simulink model "PMSM3P2LInverterCHILsystem"  (R2026a)
settings: Solver=FixedStepAuto  StopTime=inf  FixedStep=Ts_CPU  EnableMultiTasking=on
undefined symbols (not defined in the file): DiscIntNeverNeededParam, F28379D_ADC_MaxCount, F28379D_ADC_Vmax, Foc_Ki_IxTcpu, Foc_Ki_S, Foc_Kp_I, Foc_Kp_S, Ia_offset, Ib_offset, IO334, IO334_DAC_Vmax, IO334_iDAC_bias, IO334_iDAC_gain, Maxon_645604_J, Maxon_645604_lambda_pm, Maxon_645604_Ld, Maxon_645604_Lq, Maxon_645604_Np, Maxon_645604_Rs, Maxon_645604_StaticF, Maxon_645604_ViscousF, Maxon_Mile_Nslits, PMSM3P2LInverter_limited, PMSM_3P2L_Inverter_Plant, PU_System_I_base, PU_System_N_base, PWM_frequency, Ts_CAN_Tx, Ts_CPU, ts_FPGA_mdl, Ts_UI
libraries: speedgoatlib_hdlCoder_IO3xx x31, mcbcontrolslib x8, canmsglib x6, speedgoatlib_IO611 x3, mcbeeMathTransformLib x3, slpidlib x3, simulink x3, mcbpositiondecoderlib x3, pwm_cpulib x2, mcbhdlplantlib x2, demo_controls x1, quadrature_cpulib x1
(part 2 of 3)

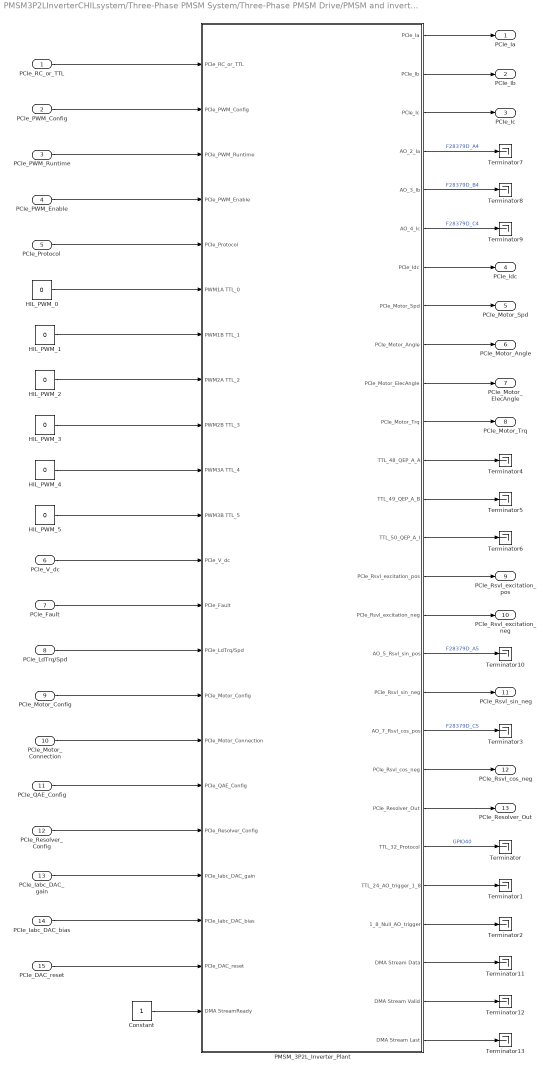
== system PMSM3P2LInverterCHILsystem/Three-Phase PMSM System/Three-Phase PMSM Drive/PMSM and inverter with switching dynamics/PMSM_3P2L_Inverter_Plant_TBR ==
  PCIe_RC_or_TTL : Inport
  PCIe_PWM_Config : Inport  Port=2
  PCIe_PWM_Runtime : Inport  Port=3
  PCIe_PWM_Enable : Inport  Port=4
  PCIe_Protocol : Inport  Port=5
  PCIe_V_dc : Inport  Port=6
  PCIe_Fault : Inport  Port=7
  PCIe_LdTrq/Spd : Inport  Port=8
  PCIe_Motor_Config : Inport  Port=9
  PCIe_Motor_Connection : Inport  Port=10
  PCIe_QAE_Config : Inport  Port=11
  PCIe_Resolver_Config : Inport  Port=12
  PCIe_Iabc_DAC_gain : Inport  Port=13
  PCIe_Iabc_DAC_bias : Inport  Port=14
  PCIe_DAC_reset : Inport  Port=15
  Constant : Constant  OutDataTypeStr=boolean
  HIL_PWM_{0..5} (6 alike) : Constant  Value=0  OutDataTypeStr=boolean
  PMSM_3P2L_Inverter_Plant : Subsystem  mask(Speedgoat IO334-325k Interface Block){module_id=1, slot=-1, ts=-1, dacGain_1=+/- 10.0V, dacActiv_1=off, dacGain_2=+/- 2.5V, dacActiv_2=on, dacGain_3=+/- 2.5V, dacActiv_3=on, dacGain_4=+/- 2.5V, dacActiv_4=on, dacGain_5=+/- 2.5V, dacActiv_5=on, dacGain_6=+/- 10.0V, dacActiv_6=off, dacGain_7=+/- 2.5V, dacActiv_7=on, dacGain_8=+/- 10.0V, dacActiv_8=off, dacGain_9=+/- 10.0V, dacActiv_9=off, dacGain_10=+/- 10.0V, dacActiv_10=off, dacGain_11=+/- 10.0V, dacActiv_11=off, dacGain_12=+/- 10.0V, dacActiv_12=off, dacGain_13=+/- 10.0V, dacActiv_13=off, dacGain_14=+/- 10.0V, dacActiv_14=off, dacGain_15=+/- 10.0V, dacActiv_15=off, dacGain_16=+/- 10.0V, dacActiv_16=off, PullRPort0=pull-up 3.3V, VioPort0=3.3V, PullRPort1=pull-up 3.3V, VioPort1=3.3V, PullRPort2=pull-up 3.3V, VioPort2=3.3V, PullRPort3=pull-up 3.3V, VioPort3=3.3V, PullRPort4=pull-up 3.3V, VioPort4=3.3V, PullRPort5=pull-up 3.3V, VioPort5=3.3V, PullRPort6=pull-up 3.3V, VioPort6=3.3V, fpga_sync_mode=on, reset_mode=on, reset_mode_stop=on, FpgaFreq=200}
      mask prompts: module_id "FPGA Module Identifier:"; slot "PCI slot (-1: autosearch):"; ts "Sample time:"; dacGain_1 "DAC Ch 01 Range"; dacActiv_1 "Active"; dacGain_2 "DAC Ch 02 Range"; dacActiv_2 "Active"; dacGain_3 "DAC Ch 03 Range"; dacActiv_3 "Active"; dacGain_4 "DAC Ch 04 Range"; dacActiv_4 "Active"; dacGain_5 "DAC Ch 05 Range"; dacActiv_5 "Active"; dacGain_6 "DAC Ch 06 Range"; dacActiv_6 "Active"; dacGain_7 "DAC Ch 07 Range"; dacActiv_7 "Active"; dacGain_8 "DAC Ch 08 Range"; dacActiv_8 "Active"; dacGain_9 "DAC Ch 09 Range"; dacActiv_9 "Active"; dacGain_10 "DAC Ch 10 Range"; dacActiv_10 "Active"; dacGain_11 "DAC Ch 11 Range"; dacActiv_11 "Active"; dacGain_12 "DAC Ch 12 Range"; dacActiv_12 "Active"; dacGain_13 "DAC Ch 13 Range"; dacActiv_13 "Active"; dacGain_14 "DAC Ch 14 Range"; dacActiv_14 "Active"; dacGain_15 "DAC Ch 15 Range"; dacActiv_15 "Active"; dacGain_16 "DAC Ch 16 Range"; dacActiv_16 "Active"; PullRPort0 "pull resistor"; VioPort0 "I/O voltage"; PullRPort1 "pull resistor"; VioPort1 "I/O voltage"; PullRPort2 "pull resistor"; VioPort2 "I/O voltage"; PullRPort3 "pull resistor"; VioPort3 "I/O voltage"; PullRPort4 "pull resistor"; VioPort4 "I/O voltage"; PullRPort5 "pull resistor"; VioPort5 "I/O voltage"; PullRPort6 "pull resistor"; VioPort6 "I/O voltage"; fpga_sync_mode "Run FPGA only when target application runs"; reset_mode "Reset FPGA states on start"; reset_mode_stop "Reset FPGA states on stop"; FpgaFreq "FPGA Frequency [MHz]"
      mask help: Simulink Real-Time Interface Block for Speedgoat IO334-325k.
      mask init:
      | hdlslrt.backend.mfpgaparameters;
      | if sg.hdlc.utils.compareMatlabVersion('~=', 'R2025a')
      | 	sg.hdlc.warning(['The interface model that you are attempting to use was generated ',...
      | 		'in MATLAB R2025a and may not be compatible with the version you are currently using. ',...
      | 		'Attempting to use this interface model in a different MATLAB release can lead to ',...
      | 		'application crashes or other unpredictable behavior. ',...
      | 		'In order to avoid this and ensure stability and correct functionality, ',...
      | 		'we highly recommend regenerating the model with your current MATLAB release.']);
      | end
      mask Help: eval('sg.hdlc.utils.help.show(''refentry_workflow_generated_model'',''isHdlcHelp'', true)')
      mask TypeOptions dacGain_1: AD5547 Setup/dacGain_1
      mask TypeOptions dacActiv_1: AD5547 Setup/dacActiv_1
      mask TypeOptions dacGain_2: AD5547 Setup/dacGain_2
      mask TypeOptions dacActiv_2: AD5547 Setup/dacActiv_2
      mask TypeOptions dacGain_3: AD5547 Setup/dacGain_3
      mask TypeOptions dacActiv_3: AD5547 Setup/dacActiv_3
      mask TypeOptions dacGain_4: AD5547 Setup/dacGain_4
      mask TypeOptions dacActiv_4: AD5547 Setup/dacActiv_4
      mask TypeOptions dacGain_5: AD5547 Setup/dacGain_5
      mask TypeOptions dacActiv_5: AD5547 Setup/dacActiv_5
      mask TypeOptions dacGain_6: AD5547 Setup/dacGain_6
      mask TypeOptions dacActiv_6: AD5547 Setup/dacActiv_6
      mask TypeOptions dacGain_7: AD5547 Setup/dacGain_7
      mask TypeOptions dacActiv_7: AD5547 Setup/dacActiv_7
      mask TypeOptions dacGain_8: AD5547 Setup/dacGain_8
      mask TypeOptions dacActiv_8: AD5547 Setup/dacActiv_8
      mask TypeOptions dacGain_9: AD5547 Setup/dacGain_9
      mask TypeOptions dacActiv_9: AD5547 Setup/dacActiv_9
      mask TypeOptions dacGain_10: AD5547 Setup/dacGain_10
      mask TypeOptions dacActiv_10: AD5547 Setup/dacActiv_10
      mask TypeOptions dacGain_11: AD5547 Setup/dacGain_11
      mask TypeOptions dacActiv_11: AD5547 Setup/dacActiv_11
      mask TypeOptions dacGain_12: AD5547 Setup/dacGain_12
      mask TypeOptions dacActiv_12: AD5547 Setup/dacActiv_12
      mask TypeOptions dacGain_13: AD5547 Setup/dacGain_13
      mask TypeOptions dacActiv_13: AD5547 Setup/dacActiv_13
      mask TypeOptions dacGain_14: AD5547 Setup/dacGain_14
      mask TypeOptions dacActiv_14: AD5547 Setup/dacActiv_14
      mask TypeOptions dacGain_15: AD5547 Setup/dacGain_15
      mask TypeOptions dacActiv_15: AD5547 Setup/dacActiv_15
      mask TypeOptions dacGain_16: AD5547 Setup/dacGain_16
      mask TypeOptions dacActiv_16: AD5547 Setup/dacActiv_16
      mask TypeOptions PullRPort0: Port Settings -2x 0x00590000/PullRPort0
      mask Callback PullRPort0: sg_fpga_HDLCoder_io3xx_2x_m(2);
      mask TypeOptions VioPort0: Port Settings -2x 0x00590000/VioPort0
      mask Callback VioPort0: sg_fpga_HDLCoder_io3xx_2x_m(2);
      mask TypeOptions PullRPort1: Port Settings -2x 0x00590000/PullRPort1
      mask Callback PullRPort1: sg_fpga_HDLCoder_io3xx_2x_m(2);
      mask TypeOptions VioPort1: Port Settings -2x 0x00590000/VioPort1
      mask Callback VioPort1: sg_fpga_HDLCoder_io3xx_2x_m(2);
      mask TypeOptions PullRPort2: Port Settings -2x 0x00590000/PullRPort2
      mask Callback PullRPort2: sg_fpga_HDLCoder_io3xx_2x_m(2);
      mask TypeOptions VioPort2: Port Settings -2x 0x00590000/VioPort2
      mask Callback VioPort2: sg_fpga_HDLCoder_io3xx_2x_m(2);
      mask TypeOptions PullRPort3: Port Settings -2x 0x00590000/PullRPort3
      mask Callback PullRPort3: sg_fpga_HDLCoder_io3xx_2x_m(2);
      mask TypeOptions VioPort3: Port Settings -2x 0x00590000/VioPort3
      mask Callback VioPort3: sg_fpga_HDLCoder_io3xx_2x_m(2);
      mask TypeOptions PullRPort4: Port Settings -2x 0x00590000/PullRPort4
      mask Callback PullRPort4: sg_fpga_HDLCoder_io3xx_2x_m(2);
      mask TypeOptions VioPort4: Port Settings -2x 0x00590000/VioPort4
      mask Callback VioPort4: sg_fpga_HDLCoder_io3xx_2x_m(2);
      mask TypeOptions PullRPort5: Port Settings -2x 0x00590000/PullRPort5
      mask Callback PullRPort5: sg_fpga_HDLCoder_io3xx_2x_m(2);
      mask TypeOptions VioPort5: Port Settings -2x 0x00590000/VioPort5
      mask Callback VioPort5: sg_fpga_HDLCoder_io3xx_2x_m(2);
      mask TypeOptions PullRPort6: Port Settings -2x 0x00590000/PullRPort6
      mask Callback PullRPort6: sg_fpga_HDLCoder_io3xx_2x_m(2);
      mask TypeOptions VioPort6: Port Settings -2x 0x00590000/VioPort6
      mask Callback VioPort6: sg_fpga_HDLCoder_io3xx_2x_m(2);
      mask TypeOptions fpga_sync_mode: IO3xx Setup/fpga_sync_mode
      mask TypeOptions reset_mode: IO3xx Setup/reset_mode
      mask TypeOptions reset_mode_stop: IO3xx Setup/reset_mode_stop
      mask DialogControl DAC Prompt: DAC
      mask DialogControl dacGrp_1 Prompt: Ch 01 to 08
      mask DialogControl dacGrp_2 Prompt: Ch 09 to 16
      mask DialogControl IO33421 Prompt: IO334-21
      mask DialogControl port1 Prompt: Port 1
      mask DialogControl port2 Prompt: Port 2
      mask DialogControl port3 Prompt: Port 3
      mask DialogControl port4 Prompt: Port 4
      mask DialogControl port5 Prompt: Port 5
      mask DialogControl port6 Prompt: Port 6
      mask DialogControl port7 Prompt: Port 7
      mask Display:
      | SetupBlkPath = sghdlc.model.findSystem(gcb, 'LookUnderMasks', 'all', 'FollowLinks', 'on', 'regexp', 'on', 'Name', 'IO3(\d|x){2}\s+Setup' );
      | SetupBlkPath = SetupBlkPath{1};
      | TS = get_param(SetupBlkPath,'timestamp_mcs');
      | disp(sprintf('Speedgoat IO334-325k\n\nTimestamp\n%s\n\nReference Design\nVersion 1.0\n\nMATLAB R2025a\n\nPCIe Link Width: X4\nTiming Severity: error\nRear Plugin: -21\nAurora Mode: None\nAurora Crc: true\nAurora Byteswap: true\nVerifier: off\nVerifier: JTAG\n', TS))
  Terminator{,1..13} (14 alike) : Terminator
  PCIe_Ia : Outport
  PCIe_Ib : Outport  Port=2
  PCIe_Ic : Outport  Port=3
  PCIe_Idc : Outport  Port=4
  PCIe_Motor_Spd : Outport  Port=5
  PCIe_Motor_Angle : Outport  Port=6
  PCIe_Motor_ElecAngle : Outport  Port=7
  PCIe_Motor_Trq : Outport  Port=8
  PCIe_Rsvl_excitation_pos : Outport  Port=9
  PCIe_Rsvl_excitation_neg : Outport  Port=10
  PCIe_Rsvl_sin_neg : Outport  Port=11
  PCIe_Rsvl_cos_neg : Outport  Port=12
  PCIe_Resolver_Out : Outport  Port=13
  wires:
  PMSM_3P2L_Inverter_Plant/1(PCIe_Ia) -> PCIe_Ia/1
  PMSM_3P2L_Inverter_Plant/3(PCIe_Ic) -> PCIe_Ic/1
  PMSM_3P2L_Inverter_Plant/2(PCIe_Ib) -> PCIe_Ib/1
  PMSM_3P2L_Inverter_Plant/7(PCIe_Idc) -> PCIe_Idc/1
  PMSM_3P2L_Inverter_Plant/8(PCIe_Motor_Spd) -> PCIe_Motor_Spd/1
  PMSM_3P2L_Inverter_Plant/9(PCIe_Motor_Angle) -> PCIe_Motor_Angle/1
  PMSM_3P2L_Inverter_Plant/10(PCIe_Motor_ElecAngle) -> PCIe_Motor_ElecAngle/1
  PMSM_3P2L_Inverter_Plant/11(PCIe_Motor_Trq) -> PCIe_Motor_Trq/1
  PMSM_3P2L_Inverter_Plant/15(PCIe_Rsvl_excitation_pos) -> PCIe_Rsvl_excitation_pos/1
  PMSM_3P2L_Inverter_Plant/16(PCIe_Rsvl_excitation_neg) -> PCIe_Rsvl_excitation_neg/1
  PMSM_3P2L_Inverter_Plant/17(AO_5_Rsvl_sin_pos) -> Terminator10/1  "F28379D_A5"
  PMSM_3P2L_Inverter_Plant/18(PCIe_Rsvl_sin_neg) -> PCIe_Rsvl_sin_neg/1
  PMSM_3P2L_Inverter_Plant/20(PCIe_Rsvl_cos_neg) -> PCIe_Rsvl_cos_neg/1
  PMSM_3P2L_Inverter_Plant/21(PCIe_Resolver_Out) -> PCIe_Resolver_Out/1
  PMSM_3P2L_Inverter_Plant/22(TTL_32_Protocol) -> Terminator/1  "GPIO40"
  PMSM_3P2L_Inverter_Plant/23(TTL_24_AO_trigger_1_8) -> Terminator1/1
  PMSM_3P2L_Inverter_Plant/24(1_8_Null_AO_trigger) -> Terminator2/1
  PMSM_3P2L_Inverter_Plant/19(AO_7_Rsvl_cos_pos) -> Terminator3/1  "F28379D_C5"
  PMSM_3P2L_Inverter_Plant/14("TTL_50_QEP_A_I   ") -> Terminator6/1
  PMSM_3P2L_Inverter_Plant/12(TTL_48_QEP_A_A) -> Terminator4/1
  PMSM_3P2L_Inverter_Plant/13(TTL_49_QEP_A_B) -> Terminator5/1
  PMSM_3P2L_Inverter_Plant/6(AO_4_Ic) -> Terminator9/1  "F28379D_C4"
  PMSM_3P2L_Inverter_Plant/4(AO_2_Ia) -> Terminator7/1  "F28379D_A4"
  PMSM_3P2L_Inverter_Plant/5(AO_3_Ib) -> Terminator8/1  "F28379D_B4"
  PCIe_RC_or_TTL/1 -> PMSM_3P2L_Inverter_Plant/1(PCIe_RC_or_TTL)
  PCIe_PWM_Config/1 -> PMSM_3P2L_Inverter_Plant/2(PCIe_PWM_Config)
  PCIe_PWM_Runtime/1 -> PMSM_3P2L_Inverter_Plant/3(PCIe_PWM_Runtime)
  PCIe_PWM_Enable/1 -> PMSM_3P2L_Inverter_Plant/4(PCIe_PWM_Enable)
  PCIe_Protocol/1 -> PMSM_3P2L_Inverter_Plant/5(PCIe_Protocol)
  HIL_PWM_0/1 -> PMSM_3P2L_Inverter_Plant/6(PWM1A TTL_0)
  HIL_PWM_1/1 -> PMSM_3P2L_Inverter_Plant/7(PWM1B TTL_1)
  HIL_PWM_2/1 -> PMSM_3P2L_Inverter_Plant/8(PWM2A TTL_2)
  HIL_PWM_3/1 -> PMSM_3P2L_Inverter_Plant/9(PWM2B TTL_3)
  HIL_PWM_4/1 -> PMSM_3P2L_Inverter_Plant/10(PWM3A TTL_4)
  HIL_PWM_5/1 -> PMSM_3P2L_Inverter_Plant/11(PWM3B TTL_5)
  PCIe_V_dc/1 -> PMSM_3P2L_Inverter_Plant/12(PCIe_V_dc)
  PCIe_Fault/1 -> PMSM_3P2L_Inverter_Plant/13(PCIe_Fault)
  PCIe_LdTrq/Spd/1 -> PMSM_3P2L_Inverter_Plant/14(PCIe_LdTrq/Spd)
  PCIe_Motor_Connection/1 -> PMSM_3P2L_Inverter_Plant/16(PCIe_Motor_Connection)
  PCIe_QAE_Config/1 -> PMSM_3P2L_Inverter_Plant/17(PCIe_QAE_Config)
  PCIe_Resolver_Config/1 -> PMSM_3P2L_Inverter_Plant/18(PCIe_Resolver_Config)
  PCIe_Iabc_DAC_gain/1 -> PMSM_3P2L_Inverter_Plant/19(PCIe_Iabc_DAC_gain)
  PCIe_Iabc_DAC_bias/1 -> PMSM_3P2L_Inverter_Plant/20(PCIe_Iabc_DAC_bias)
  PCIe_DAC_reset/1 -> PMSM_3P2L_Inverter_Plant/21(PCIe_DAC_reset)
  PCIe_Motor_Config/1 -> PMSM_3P2L_Inverter_Plant/15(PCIe_Motor_Config)
  PMSM_3P2L_Inverter_Plant/26(DMA Stream Valid) -> Terminator12/1
  PMSM_3P2L_Inverter_Plant/25(DMA Stream Data) -> Terminator11/1
  PMSM_3P2L_Inverter_Plant/27(DMA Stream Last) -> Terminator13/1
  Constant/1 -> PMSM_3P2L_Inverter_Plant/22(DMA StreamReady)

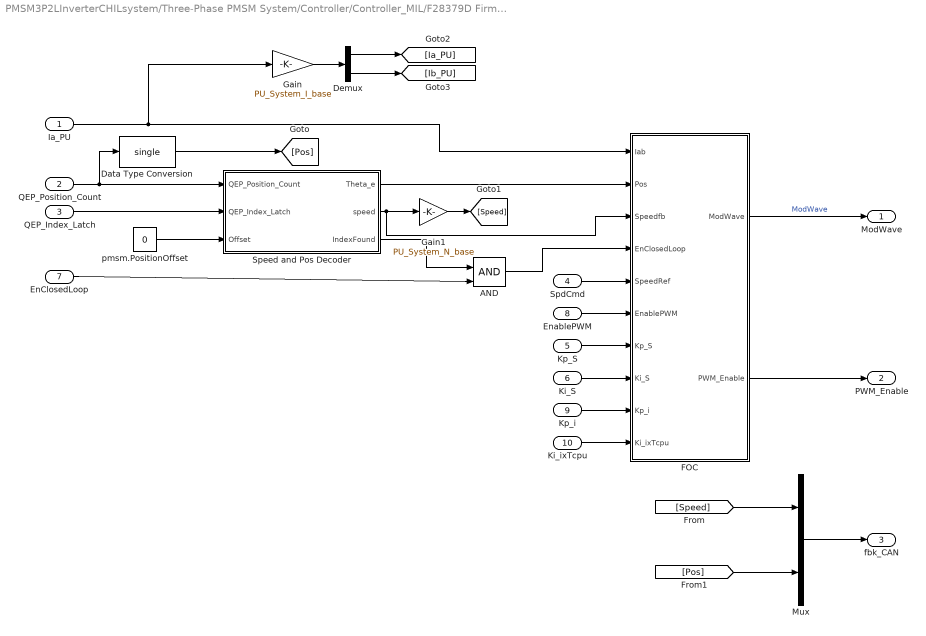
== system PMSM3P2LInverterCHILsystem/Three-Phase PMSM System/Controller/Controller_MIL/F28379D Firmware/Controller Algorithm ==
  Ia_PU : Inport
  QEP_Position_Count : Inport  Port=2
  QEP_Index_Latch : Inport  Port=3
  SpdCmd : Inport  Port=4
  Kp_S : Inport  Port=5
  Ki_S : Inport  Port=6
  EnClosedLoop : Inport  Port=7
  EnablePWM : Inport  Port=8
  Kp_i : Inport  Port=9
  Ki_ixTcpu : Inport  Port=10
  AND : Logic  IconShape=distinctive  AllPortsSameDT=off  OutDataTypeStr=boolean
  Data Type Conversion : DataTypeConversion  OutDataTypeStr=single  SaturateOnIntegerOverflow=off  RndMeth=Floor
  Demux : Demux  Outputs=2
  FOC : Subsystem
  Gain : Gain  Gain=PU_System_I_base
  Gain1 : Gain  Gain=PU_System_N_base
  Mux : Mux  Inputs=2
  Speed and Pos Decoder : Subsystem
  pmsm.PositionOffset : Constant  Value=0  SampleTime=-1
  ModWave : Outport
  PWM_Enable : Outport  Port=2
  fbk_CAN : Outport  Port=3
  wires:
  EnClosedLoop/1 -> AND/2
  Speed and Pos Decoder/1(Theta_e) -> FOC/2(Pos)
  Ia_PU/1 -> FOC/1(Iab), Gain/1
  EnablePWM/1 -> FOC/6(EnablePWM)
  Speed and Pos Decoder/3(IndexFound) -> AND/1
  AND/1 -> FOC/4(EnClosedLoop)
  pmsm.PositionOffset/1 -> Speed and Pos Decoder/3(Offset)
  Speed and Pos Decoder/2(speed) -> FOC/3(Speedfb), Gain1/1
  FOC/2(PWM_Enable) -> PWM_Enable/1
  QEP_Index_Latch/1 -> Speed and Pos Decoder/2(QEP_Index_Latch)
  FOC/1(ModWave) -> ModWave/1  "ModWave"
  Kp_S/1 -> FOC/7(Kp_S)
  Ki_S/1 -> FOC/8(Ki_S)
  SpdCmd/1 -> FOC/5(SpeedRef)
  [Speed] -> Mux/1
  [Pos] -> Mux/2
  Mux/1 -> fbk_CAN/1
  Demux/1 -> [Ia_PU]
  Demux/2 -> [Ib_PU]
  Kp_i/1 -> FOC/9(Kp_i)
  Ki_ixTcpu/1 -> FOC/10(Ki_ixTcpu)
  Gain/1 -> Demux/1
  Gain1/1 -> [Speed]
  QEP_Position_Count/1 -> Speed and Pos Decoder/1(QEP_Position_Count), Data Type Conversion/1
  Data Type Conversion/1 -> [Pos]

== system PMSM3P2LInverterCHILsystem/Three-Phase PMSM System/Controller/Controller_MIL/F28379D Firmware/Phase_Current_Rescaling ==
  Ia_ADC : Inport
  Ib_ADC : Inport  Port=2
  IaOffset : Inport  Port=3
  IbOffset : Inport  Port=4
  ADCtoA : Gain  Gain=10/IO334_DAC_Vmax/IO334_iDAC_gain  RndMeth=Simplest  OutDataTypeStr=Inherit: Same as input
  Add : Sum  Inputs=+-
  Add Constant : Bias  Bias=-2^11*IO334_DAC_Vmax/F28379D_ADC_Vmax  SaturateOnIntegerOverflow=off
  Get ADC Voltage : Gain  Gain=F28379D_ADC_Vmax/F28379D_ADC_MaxCount  OutDataTypeStr=single  RndMeth=Simplest
  Mux : Mux  Inputs=2
  Mux1 : Mux  Inputs=2
  PU_Conversion : Gain  Gain=1/PU_System_I_base  RndMeth=Simplest  OutDataTypeStr=Inherit: Same as input
  Rate Transition : RateTransition
  Iab_meas_PU : Outport  VectorParamsAs1DForOutWhenUnconnected=off
  wires:
  Mux1/1 -> Rate Transition/1
  Ia_ADC/1 -> Mux/1
  Ib_ADC/1 -> Mux/2
  Mux/1 -> Add Constant/1
  PU_Conversion/1 -> Iab_meas_PU/1
  IaOffset/1 -> Mux1/1
  IbOffset/1 -> Mux1/2
  Add Constant/1 -> Get ADC Voltage/1
  Get ADC Voltage/1 -> ADCtoA/1  "Currents_inDACvoltages"
  Rate Transition/1 -> Add/2
  ADCtoA/1 -> Add/1  "Currents_A"
  Add/1 -> PU_Conversion/1  "Currents_no_offset"

== system PMSM3P2LInverterCHILsystem/Three-Phase PMSM System/Controller/Controller_MIL/F28379D Firmware/Speed Conditioning ==
  Spd[rpm] : Inport
  hz2pu : Gain  Gain=60/(PU_System_N_base *Maxon_645604_Np)  RndMeth=Simplest  OutDataTypeStr=Inherit: Same as input
  rads2hz : Gain  Gain=Maxon_645604_Np/(2*pi)
  rmp2rads : Gain  Gain=2*pi/60
  Spd[PU] : Outport
  wires:
  Spd[rpm]/1 -> rmp2rads/1
  rmp2rads/1 -> rads2hz/1
  rads2hz/1 -> hz2pu/1
  hz2pu/1 -> Spd[PU]/1

== system PMSM3P2LInverterCHILsystem/Three-Phase PMSM System/Three-Phase PMSM Drive/PMSM and average inverter/Encoder Simulation/Get_PU  ==
  rad : Inport
  Constant2 : Constant  Value=2*pi  OutDataTypeStr=single  SampleTime=-1
  Get_PU : Gain  Gain=1/(2*pi)  RndMeth=Simplest  OutDataTypeStr=Inherit: Same as input
  Mod : Math  Operator=mod
  PU : Outport  VectorParamsAs1DForOutWhenUnconnected=off
  wires:
  Get_PU/1 -> PU/1
  Mod/1 -> Get_PU/1
  Constant2/1 -> Mod/2
  rad/1 -> Mod/1

== system PMSM3P2LInverterCHILsystem/Three-Phase PMSM System/Three-Phase PMSM Drive/PMSM and average inverter/Encoder Simulation/Wrap ==
  in : Inport
  Constant2 : Constant  OutDataTypeStr=single  SampleTime=-1
  Mod : Math  Operator=mod
  out : Outport  VectorParamsAs1DForOutWhenUnconnected=off
  wires:
  Mod/1 -> out/1
  Constant2/1 -> Mod/2
  in/1 -> Mod/1

== system PMSM3P2LInverterCHILsystem/Three-Phase PMSM System/Three-Phase PMSM Drive/PMSM and average inverter/Runtime to DC/To Dc A1 ==
  A_on : Inport
  A_off : Inport  Port=2
  Add : Sum
  Add Constant1 : Bias  Bias=1  SaturateOnIntegerOverflow=off
  Data Type Conversion3 : DataTypeConversion  OutDataTypeStr=double  SaturateOnIntegerOverflow=off  RndMeth=Floor
  Data Type Conversion5 : DataTypeConversion  OutDataTypeStr=double  SaturateOnIntegerOverflow=off  RndMeth=Floor
  Divide : Product  Inputs=*/
  Gain1 : Gain  Gain=-2
  Dc : Outport
  wires:
  Data Type Conversion5/1 -> Add/2
  Add Constant1/1 -> Dc/1
  Gain1/1 -> Add Constant1/1
  Add/1 -> Divide/2
  Data Type Conversion3/1 -> Add/1, Divide/1
  A_off/1 -> Data Type Conversion5/1
  Divide/1 -> Gain1/1
  A_on/1 -> Data Type Conversion3/1

== system PMSM3P2LInverterCHILsystem/Three-Phase PMSM System/Three-Phase PMSM Drive/PMSM and average inverter/Runtime to DC/To Dc A2 ==
  A_on : Inport
  A_off : Inport  Port=2
  Add : Sum
  Add Constant1 : Bias  Bias=1  SaturateOnIntegerOverflow=off
  Data Type Conversion3 : DataTypeConversion  OutDataTypeStr=double  SaturateOnIntegerOverflow=off  RndMeth=Floor
  Data Type Conversion5 : DataTypeConversion  OutDataTypeStr=double  SaturateOnIntegerOverflow=off  RndMeth=Floor
  Divide : Product  Inputs=*/
  Gain1 : Gain  Gain=-2
  Dc : Outport
  wires:
  A_on/1 -> Data Type Conversion3/1
  Divide/1 -> Gain1/1
  A_off/1 -> Data Type Conversion5/1
  Data Type Conversion3/1 -> Divide/1, Add/1
  Add/1 -> Divide/2
  Gain1/1 -> Add Constant1/1
  Add Constant1/1 -> Dc/1
  Data Type Conversion5/1 -> Add/2

== system PMSM3P2LInverterCHILsystem/Three-Phase PMSM System/Three-Phase PMSM Drive/PMSM and average inverter/Runtime to DC/To Dc A3 ==
  A_on : Inport
  A_off : Inport  Port=2
  Add : Sum
  Add Constant1 : Bias  Bias=1  SaturateOnIntegerOverflow=off
  Data Type Conversion3 : DataTypeConversion  OutDataTypeStr=double  SaturateOnIntegerOverflow=off  RndMeth=Floor
  Data Type Conversion5 : DataTypeConversion  OutDataTypeStr=double  SaturateOnIntegerOverflow=off  RndMeth=Floor
  Divide : Product  Inputs=*/
  Gain1 : Gain  Gain=-2
  Dc : Outport
  wires:
  Data Type Conversion5/1 -> Add/2
  Add Constant1/1 -> Dc/1
  Gain1/1 -> Add Constant1/1
  Add/1 -> Divide/2
  Data Type Conversion3/1 -> Add/1, Divide/1
  A_off/1 -> Data Type Conversion5/1
  Divide/1 -> Gain1/1
  A_on/1 -> Data Type Conversion3/1

== system PMSM3P2LInverterCHILsystem/Three-Phase PMSM System/Three-Phase PMSM Drive/PMSM and inverter with switching dynamics/DAC Config/Subsystem ==
  Plant_frequency : Inport
  SignalFrequency : Inport  Port=2
  Add : Sum  Inputs=+-
  Data Type Conversion : DataTypeConversion  OutDataTypeStr=uint16  SaturateOnIntegerOverflow=off  RndMeth=Floor
  Divide : Product  Inputs=*/
  constant : Constant  VectorParams1D=off  SampleTime=-1
  DAC_reset : Outport
  wires:
  SignalFrequency/1 -> Divide/2
  Add/1 -> Data Type Conversion/1
  Divide/1 -> Add/1
  Data Type Conversion/1 -> DAC_reset/1
  constant/1 -> Add/2
  Plant_frequency/1 -> Divide/1

== system PMSM3P2LInverterCHILsystem/Three-Phase PMSM System/Three-Phase PMSM Drive/PMSM and inverter with switching dynamics/Encoder Simulation/Get_PU  ==
  rad : Inport
  Constant2 : Constant  Value=2*pi  OutDataTypeStr=single  SampleTime=-1
  Get_PU : Gain  Gain=1/(2*pi)  RndMeth=Simplest  OutDataTypeStr=Inherit: Same as input
  Mod : Math  Operator=mod
  PU : Outport  VectorParamsAs1DForOutWhenUnconnected=off
  wires:
  Get_PU/1 -> PU/1
  Mod/1 -> Get_PU/1
  Constant2/1 -> Mod/2
  rad/1 -> Mod/1

== system PMSM3P2LInverterCHILsystem/Three-Phase PMSM System/Three-Phase PMSM Drive/PMSM and inverter with switching dynamics/Encoder Simulation/Wrap ==
  in : Inport
  Constant2 : Constant  OutDataTypeStr=single  SampleTime=-1
  Mod : Math  Operator=mod
  out : Outport  VectorParamsAs1DForOutWhenUnconnected=off
  wires:
  Mod/1 -> out/1
  Constant2/1 -> Mod/2
  in/1 -> Mod/1

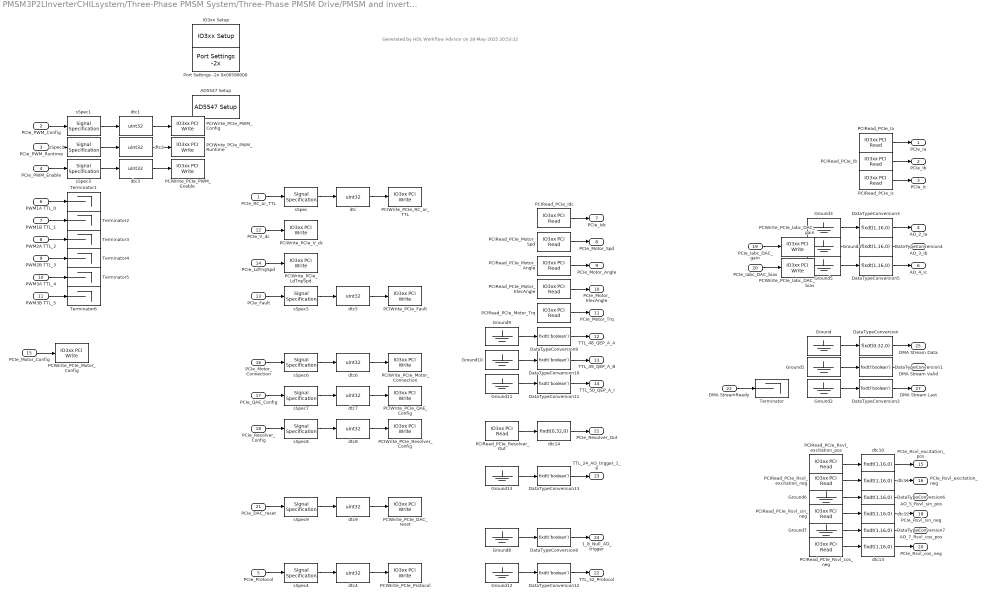
== system PMSM3P2LInverterCHILsystem/Three-Phase PMSM System/Three-Phase PMSM Drive/PMSM and inverter with switching dynamics/PMSM_3P2L_Inverter_Plant_TBR/PMSM_3P2L_Inverter_Plant ==
  note: Generated by HDL Workflow Advisor on 28-May-2025 20:53:32
  PCIe_RC_or_TTL : Inport
  PCIe_PWM_Config : Inport  Port=2
  PCIe_PWM_Runtime : Inport  Port=3
  PCIe_PWM_Enable : Inport  Port=4
  PCIe_Protocol : Inport  Port=5
  PWM1A TTL_0 : Inport  Port=6
  PWM1B TTL_1 : Inport  Port=7
  PWM2A TTL_2 : Inport  Port=8
  PWM2B TTL_3 : Inport  Port=9
  PWM3A TTL_4 : Inport  Port=10
  PWM3B TTL_5 : Inport  Port=11
  PCIe_V_dc : Inport  Port=12
  PCIe_Fault : Inport  Port=13
  PCIe_LdTrq/Spd : Inport  Port=14
  PCIe_Motor_Config : Inport  Port=15
  PCIe_Motor_Connection : Inport  Port=16
  PCIe_QAE_Config : Inport  Port=17
  PCIe_Resolver_Config : Inport  Port=18
  PCIe_Iabc_DAC_gain : Inport  Port=19
  PCIe_Iabc_DAC_bias : Inport  Port=20
  PCIe_DAC_reset : Inport  Port=21
  DMA StreamReady : Inport  Port=22
  AD5547 Setup : speedgoatlib_hdlCoder_IO3xx/AD5547 Setup  module_id=module_id  dacReset=on  dacGain_1=+/- 10.0V  dacActiv_1=off  dacInit_1=0  dacGain_2=+/- 2.5V  dacActiv_2=on  dacInit_2=0  dacGain_3=+/- 2.5V  dacActiv_3=on  dacInit_3=0  dacGain_4=+/- 2.5V  dacActiv_4=on  dacInit_4=0  dacGain_5=+/- 2.5V  dacActiv_5=on  dacInit_5=0  dacGain_6=+/- 10.0V  dacActiv_6=off  dacInit_6=0  dacGain_7=+/- 2.5V  dacActiv_7=on  dacInit_7=0  dacGain_8=+/- 10.0V  dacActiv_8=off  dacInit_8=0  dacGain_9=+/- 10.0V  dacActiv_9=off  dacInit_9=0  dacGain_10=+/- 10.0V  dacActiv_10=off  dacInit_10=0  dacGain_11=+/- 10.0V  dacActiv_11=off  dacInit_11=0  dacGain_12=+/- 10.0V  dacActiv_12=off  dacInit_12=0  dacGain_13=+/- 10.0V  dacActiv_13=off  dacInit_13=0  dacGain_14=+/- 10.0V  dacActiv_14=off  dacInit_14=0  dacGain_15=+/- 10.0V  dacActiv_15=off  dacInit_15=0  dacGain_16=+/- 10.0V  dacActiv_16=off  dacInit_16=0  dacGain_17=+/- 10.0V  dacActiv_17=off  dacInit_17=0  dacGain_18=+/- 10.0V  dacActiv_18=off  dacInit_18=0  dacGain_19=+/- 10.0V  dacActiv_19=off  dacInit_19=0  dacGain_20=+/- 10.0V  dacActiv_20=off  dacInit_20=0  dacGain_21=+/- 10.0V  dacActiv_21=off  dacInit_21=0  dacGain_22=+/- 10.0V  dacActiv_22=off  dacInit_22=0  dacGain_23=+/- 10.0V  dacActiv_23=off  dacInit_23=0  dacGain_24=+/- 10.0V  dacActiv_24=off  dacInit_24=0  dacGain_25=+/- 10.0V  dacActiv_25=off  dacInit_25=0  dacGain_26=+/- 10.0V  dacActiv_26=off  dacInit_26=0  dacGain_27=+/- 10.0V  dacActiv_27=off  dacInit_27=0  dacGain_28=+/- 10.0V  dacActiv_28=off  dacInit_28=0  dacGain_29=+/- 10.0V  dacActiv_29=off  dacInit_29=0  dacGain_30=+/- 10.0V  dacActiv_30=off  dacInit_30=0  dacGain_31=+/- 10.0V  dacActiv_31=off  dacInit_31=0  dacGain_32=+/- 10.0V  dacActiv_32=off  dacInit_32=0
  DataTypeConversion : DataTypeConversion  OutDataTypeStr=fixdt(0,32,0)  ConvertRealWorld=Stored Integer (SI)  SaturateOnIntegerOverflow=off  RndMeth=Floor
  DataTypeConversion{1..2,8..13} (8 alike) : DataTypeConversion  OutDataTypeStr=fixdt('boolean')  ConvertRealWorld=Stored Integer (SI)  SaturateOnIntegerOverflow=off  RndMeth=Floor
  DataTypeConversion{3..7} (5 alike) : DataTypeConversion  OutDataTypeStr=fixdt(1,16,0)  ConvertRealWorld=Stored Integer (SI)  SaturateOnIntegerOverflow=off  RndMeth=Floor
  Ground{,1..13} (14 alike) : Ground
  IO3xx Setup : speedgoatlib_hdlCoder_IO3xx/IO3xx Setup  mdl_ss_name=PMSM3P2LInverter_limited/PMSM_3P2L_Inverter_Plant  board_type=IO334-325k  fpga_sync_mode=on  reset_mode=on  reset_mode_stop=on  device_id=1  module_id=module_id  pci_slot=slot  fpga_mat_file=c:\hdl_prj\hdlsrc\PMSM3P2LInverter_limited\PMSM_3P2L_Inverter_Plant.mat  timestamp_mcs=05/28/25 20:27:22  timestamp=3803399894  tsreg=hex2dec('8')  bsf_file=PMSM_3P2L_Inverter_Plant_2505281921.mcs  mcs=0  init_reg_list=[]
  PCIRead_PCIe_Ia : speedgoatlib_hdlCoder_IO3xx/IO3xx PCI Read  device_id=1  module_id=module_id  board_type=IO334-325k  port_name=PCIe_Ia  port_offset=hex2dec('128')  port_type=single  port_dim=1  strobe=0  sample_time=ts
  PCIRead_PCIe_Ib : speedgoatlib_hdlCoder_IO3xx/IO3xx PCI Read  device_id=1  module_id=module_id  board_type=IO334-325k  port_name=PCIe_Ib  port_offset=hex2dec('12C')  port_type=single  port_dim=1  strobe=0  sample_time=ts
  PCIRead_PCIe_Ic : speedgoatlib_hdlCoder_IO3xx/IO3xx PCI Read  device_id=1  module_id=module_id  board_type=IO334-325k  port_name=PCIe_Ic  port_offset=hex2dec('130')  port_type=single  port_dim=1  strobe=0  sample_time=ts
  PCIRead_PCIe_Idc : speedgoatlib_hdlCoder_IO3xx/IO3xx PCI Read  device_id=1  module_id=module_id  board_type=IO334-325k  port_name=PCIe_Idc  port_offset=hex2dec('134')  port_type=single  port_dim=1  strobe=0  sample_time=ts
  PCIRead_PCIe_Motor_Angle : speedgoatlib_hdlCoder_IO3xx/IO3xx PCI Read  device_id=1  module_id=module_id  board_type=IO334-325k  port_name=PCIe_Motor_Angle  port_offset=hex2dec('13C')  port_type=single  port_dim=1  strobe=0  sample_time=ts
  PCIRead_PCIe_Motor_ElecAngle : speedgoatlib_hdlCoder_IO3xx/IO3xx PCI Read  device_id=1  module_id=module_id  board_type=IO334-325k  port_name=PCIe_Motor_ElecAngle  port_offset=hex2dec('184')  port_type=single  port_dim=1  strobe=0  sample_time=ts
  PCIRead_PCIe_Motor_Spd : speedgoatlib_hdlCoder_IO3xx/IO3xx PCI Read  device_id=1  module_id=module_id  board_type=IO334-325k  port_name=PCIe_Motor_Spd  port_offset=hex2dec('138')  port_type=single  port_dim=1  strobe=0  sample_time=ts
  PCIRead_PCIe_Motor_Trq : speedgoatlib_hdlCoder_IO3xx/IO3xx PCI Read  device_id=1  module_id=module_id  board_type=IO334-325k  port_name=PCIe_Motor_Trq  port_offset=hex2dec('188')  port_type=single  port_dim=1  strobe=0  sample_time=ts
  PCIRead_PCIe_Resolver_Out : speedgoatlib_hdlCoder_IO3xx/IO3xx PCI Read  device_id=1  module_id=module_id  board_type=IO334-325k  port_name=PCIe_Resolver_Out  port_offset=hex2dec('1D0')  port_type=uint32  port_dim=3  strobe=hex2dec('1E0')  sample_time=ts
  PCIRead_PCIe_Rsvl_cos_neg : speedgoatlib_hdlCoder_IO3xx/IO3xx PCI Read  device_id=1  module_id=module_id  board_type=IO334-325k  port_name=PCIe_Rsvl_cos_neg  port_offset=hex2dec('198')  port_type=uint32  port_dim=1  strobe=0  sample_time=ts
  PCIRead_PCIe_Rsvl_excitation_neg : speedgoatlib_hdlCoder_IO3xx/IO3xx PCI Read  device_id=1  module_id=module_id  board_type=IO334-325k  port_name=PCIe_Rsvl_excitation_neg  port_offset=hex2dec('190')  port_type=uint32  port_dim=1  strobe=0  sample_time=ts
  PCIRead_PCIe_Rsvl_excitation_pos : speedgoatlib_hdlCoder_IO3xx/IO3xx PCI Read  device_id=1  module_id=module_id  board_type=IO334-325k  port_name=PCIe_Rsvl_excitation_pos  port_offset=hex2dec('194')  port_type=uint32  port_dim=1  strobe=0  sample_time=ts
  PCIRead_PCIe_Rsvl_sin_neg : speedgoatlib_hdlCoder_IO3xx/IO3xx PCI Read  device_id=1  module_id=module_id  board_type=IO334-325k  port_name=PCIe_Rsvl_sin_neg  port_offset=hex2dec('18C')  port_type=uint32  port_dim=1  strobe=0  sample_time=ts
  PCIWrite_PCIe_DAC_reset : speedgoatlib_hdlCoder_IO3xx/IO3xx PCI Write  device_id=1  module_id=module_id  board_type=IO334-325k  port_name=PCIe_DAC_reset  port_offset=hex2dec('124')  port_type=uint32  port_dim=1  strobe=0  sample_time=ts
  PCIWrite_PCIe_Fault : speedgoatlib_hdlCoder_IO3xx/IO3xx PCI Write  device_id=1  module_id=module_id  board_type=IO334-325k  port_name=PCIe_Fault  port_offset=hex2dec('110')  port_type=uint32  port_dim=1  strobe=0  sample_time=ts
  PCIWrite_PCIe_Iabc_DAC_bias : speedgoatlib_hdlCoder_IO3xx/IO3xx PCI Write  device_id=1  module_id=module_id  board_type=IO334-325k  port_name=PCIe_Iabc_DAC_bias  port_offset=hex2dec('120')  port_type=single  port_dim=1  strobe=0  sample_time=ts
  PCIWrite_PCIe_Iabc_DAC_gain : speedgoatlib_hdlCoder_IO3xx/IO3xx PCI Write  device_id=1  module_id=module_id  board_type=IO334-325k  port_name=PCIe_Iabc_DAC_gain  port_offset=hex2dec('11C')  port_type=single  port_dim=1  strobe=0  sample_time=ts
  PCIWrite_PCIe_LdTrq/Spd : speedgoatlib_hdlCoder_IO3xx/IO3xx PCI Write  device_id=1  module_id=module_id  board_type=IO334-325k  port_name=PCIe_LdTrq//Spd  port_offset=hex2dec('114')  port_type=single  port_dim=1  strobe=0  sample_time=ts
  PCIWrite_PCIe_Motor_Config : speedgoatlib_hdlCoder_IO3xx/IO3xx PCI Write  device_id=1  module_id=module_id  board_type=IO334-325k  port_name=PCIe_Motor_Config  port_offset=hex2dec('340')  port_type=single  port_dim=9  strobe=hex2dec('380')  sample_time=ts
  PCIWrite_PCIe_Motor_Connection : speedgoatlib_hdlCoder_IO3xx/IO3xx PCI Write  device_id=1  module_id=module_id  board_type=IO334-325k  port_name=PCIe_Motor_Connection  port_offset=hex2dec('118')  port_type=uint32  port_dim=1  strobe=0  sample_time=ts
  PCIWrite_PCIe_PWM_Config : speedgoatlib_hdlCoder_IO3xx/IO3xx PCI Write  device_id=1  module_id=module_id  board_type=IO334-325k  port_name=PCIe_PWM_Config  port_offset=hex2dec('200')  port_type=uint32  port_dim=48  strobe=hex2dec('300')  sample_time=ts
  PCIWrite_PCIe_PWM_Enable : speedgoatlib_hdlCoder_IO3xx/IO3xx PCI Write  device_id=1  module_id=module_id  board_type=IO334-325k  port_name=PCIe_PWM_Enable  port_offset=hex2dec('104')  port_type=uint32  port_dim=1  strobe=0  sample_time=ts
  PCIWrite_PCIe_PWM_Runtime : speedgoatlib_hdlCoder_IO3xx/IO3xx PCI Write  device_id=1  module_id=module_id  board_type=IO334-325k  port_name=PCIe_PWM_Runtime  port_offset=hex2dec('140')  port_type=uint32  port_dim=15  strobe=hex2dec('180')  sample_time=ts
  PCIWrite_PCIe_Protocol : speedgoatlib_hdlCoder_IO3xx/IO3xx PCI Write  device_id=1  module_id=module_id  board_type=IO334-325k  port_name=PCIe_Protocol  port_offset=hex2dec('108')  port_type=uint32  port_dim=1  strobe=0  sample_time=ts
  PCIWrite_PCIe_QAE_Config : speedgoatlib_hdlCoder_IO3xx/IO3xx PCI Write  device_id=1  module_id=module_id  board_type=IO334-325k  port_name=PCIe_QAE_Config  port_offset=hex2dec('3C0')  port_type=uint32  port_dim=8  strobe=hex2dec('3E0')  sample_time=ts
  PCIWrite_PCIe_RC_or_TTL : speedgoatlib_hdlCoder_IO3xx/IO3xx PCI Write  device_id=1  module_id=module_id  board_type=IO334-325k  port_name=PCIe_RC_or_TTL  port_offset=hex2dec('100')  port_type=uint32  port_dim=1  strobe=0  sample_time=ts
  PCIWrite_PCIe_Resolver_Config : speedgoatlib_hdlCoder_IO3xx/IO3xx PCI Write  device_id=1  module_id=module_id  board_type=IO334-325k  port_name=PCIe_Resolver_Config  port_offset=hex2dec('480')  port_type=uint32  port_dim=17  strobe=hex2dec('500')  sample_time=ts
  PCIWrite_PCIe_V_dc : speedgoatlib_hdlCoder_IO3xx/IO3xx PCI Write  device_id=1  module_id=module_id  board_type=IO334-325k  port_name=PCIe_V_dc  port_offset=hex2dec('10C')  port_type=single  port_dim=1  strobe=0  sample_time=ts
  Port Settings -2x 0x00590000 : speedgoatlib_hdlCoder_IO3xx/Port Settings -2x  module_id=module_id  rearIO=-21  PullRPort0=pull-up 3.3V  VioPort0=3.3V  PullRPort1=pull-up 3.3V  VioPort1=3.3V  PullRPort2=pull-up 3.3V  VioPort2=3.3V  PullRPort3=pull-up 3.3V  VioPort3=3.3V  PullRPort4=pull-up 3.3V  VioPort4=3.3V  PullRPort5=pull-up 3.3V  VioPort5=3.3V  PullRPort6=pull-up 3.3V  VioPort6=3.3V  I2cAddrOffset=5832704  DutAddrOffset=120
  Terminator{,1..6} (7 alike) : Terminator
  dtc{,1..9} (10 alike) : DataTypeConversion  OutDataTypeStr=uint32  ConvertRealWorld=Stored Integer (SI)  SaturateOnIntegerOverflow=off
  dtc{10..13} (4 alike) : DataTypeConversion  OutDataTypeStr=fixdt(1,16,0)  ConvertRealWorld=Stored Integer (SI)  SaturateOnIntegerOverflow=off
  dtc14 : DataTypeConversion  OutDataTypeStr=fixdt(0,32,0)  ConvertRealWorld=Stored Integer (SI)  SaturateOnIntegerOverflow=off
  sSpec{,3..4,6} (4 alike) : SignalSpecification  OutDataTypeStr=fixdt('boolean')
  sSpec{1..2,5,7..8} (5 alike) : SignalSpecification  OutDataTypeStr=fixdt(0,32,0)
  sSpec9 : SignalSpecification  OutDataTypeStr=fixdt(0,16,0)
  PCIe_Ia : Outport
  PCIe_Ib : Outport  Port=2
  PCIe_Ic : Outport  Port=3
  AO_2_Ia : Outport  Port=4
  AO_3_Ib : Outport  Port=5
  AO_4_Ic : Outport  Port=6
  PCIe_Idc : Outport  Port=7
  PCIe_Motor_Spd : Outport  Port=8
  PCIe_Motor_Angle : Outport  Port=9
  PCIe_Motor_ElecAngle : Outport  Port=10
  PCIe_Motor_Trq : Outport  Port=11
  TTL_48_QEP_A_A : Outport  Port=12
  TTL_49_QEP_A_B : Outport  Port=13
  "TTL_50_QEP_A_I   " : Outport  Port=14
  PCIe_Rsvl_excitation_pos : Outport  Port=15
  PCIe_Rsvl_excitation_neg : Outport  Port=16
  AO_5_Rsvl_sin_pos : Outport  Port=17
  PCIe_Rsvl_sin_neg : Outport  Port=18
  AO_7_Rsvl_cos_pos : Outport  Port=19
  PCIe_Rsvl_cos_neg : Outport  Port=20
  PCIe_Resolver_Out : Outport  Port=21
  TTL_32_Protocol : Outport  Port=22
  TTL_24_AO_trigger_1_8 : Outport  Port=23
  1_8_Null_AO_trigger : Outport  Port=24
  DMA Stream Data : Outport  Port=25
  DMA Stream Valid : Outport  Port=26
  DMA Stream Last : Outport  Port=27
  wires:
  PCIe_RC_or_TTL/1 -> sSpec/1
  sSpec/1 -> dtc/1
  dtc/1 -> PCIWrite_PCIe_RC_or_TTL/1
  PCIe_PWM_Config/1 -> sSpec1/1
  sSpec1/1 -> dtc1/1
  dtc1/1 -> PCIWrite_PCIe_PWM_Config/1
  PCIe_PWM_Runtime/1 -> sSpec2/1
  sSpec2/1 -> dtc2/1
  dtc2/1 -> PCIWrite_PCIe_PWM_Runtime/1
  PCIe_PWM_Enable/1 -> sSpec3/1
  sSpec3/1 -> dtc3/1
  dtc3/1 -> PCIWrite_PCIe_PWM_Enable/1
  PCIe_Protocol/1 -> sSpec4/1
  sSpec4/1 -> dtc4/1
  dtc4/1 -> PCIWrite_PCIe_Protocol/1
  PCIe_V_dc/1 -> PCIWrite_PCIe_V_dc/1
  PCIe_Fault/1 -> sSpec5/1
  sSpec5/1 -> dtc5/1
  dtc5/1 -> PCIWrite_PCIe_Fault/1
  PCIe_LdTrq/Spd/1 -> PCIWrite_PCIe_LdTrq/Spd/1
  PCIe_Motor_Config/1 -> PCIWrite_PCIe_Motor_Config/1
  PCIe_Motor_Connection/1 -> sSpec6/1
  sSpec6/1 -> dtc6/1
  dtc6/1 -> PCIWrite_PCIe_Motor_Connection/1
  PCIe_QAE_Config/1 -> sSpec7/1
  sSpec7/1 -> dtc7/1
  dtc7/1 -> PCIWrite_PCIe_QAE_Config/1
  PCIe_Resolver_Config/1 -> sSpec8/1
  sSpec8/1 -> dtc8/1
  dtc8/1 -> PCIWrite_PCIe_Resolver_Config/1
  PCIe_Iabc_DAC_gain/1 -> PCIWrite_PCIe_Iabc_DAC_gain/1
  PCIe_Iabc_DAC_bias/1 -> PCIWrite_PCIe_Iabc_DAC_bias/1
  PCIe_DAC_reset/1 -> sSpec9/1
  sSpec9/1 -> dtc9/1
  dtc9/1 -> PCIWrite_PCIe_DAC_reset/1
  PCIRead_PCIe_Ia/1 -> PCIe_Ia/1
  PCIRead_PCIe_Ib/1 -> PCIe_Ib/1
  PCIRead_PCIe_Ic/1 -> PCIe_Ic/1
  PCIRead_PCIe_Idc/1 -> PCIe_Idc/1
  PCIRead_PCIe_Motor_Spd/1 -> PCIe_Motor_Spd/1
  PCIRead_PCIe_Motor_Angle/1 -> PCIe_Motor_Angle/1
  PCIRead_PCIe_Motor_ElecAngle/1 -> PCIe_Motor_ElecAngle/1
  PCIRead_PCIe_Motor_Trq/1 -> PCIe_Motor_Trq/1
  dtc10/1 -> PCIe_Rsvl_excitation_pos/1
  PCIRead_PCIe_Rsvl_excitation_pos/1 -> dtc10/1
  dtc11/1 -> PCIe_Rsvl_excitation_neg/1
  PCIRead_PCIe_Rsvl_excitation_neg/1 -> dtc11/1
  dtc12/1 -> PCIe_Rsvl_sin_neg/1
  PCIRead_PCIe_Rsvl_sin_neg/1 -> dtc12/1
  dtc13/1 -> PCIe_Rsvl_cos_neg/1
  PCIRead_PCIe_Rsvl_cos_neg/1 -> dtc13/1
  dtc14/1 -> PCIe_Resolver_Out/1
  PCIRead_PCIe_Resolver_Out/1 -> dtc14/1
  DMA StreamReady/1 -> Terminator/1
  DataTypeConversion/1 -> DMA Stream Data/1
  Ground/1 -> DataTypeConversion/1
  DataTypeConversion1/1 -> DMA Stream Valid/1
  Ground1/1 -> DataTypeConversion1/1
  DataTypeConversion2/1 -> DMA Stream Last/1
  Ground2/1 -> DataTypeConversion2/1
  DataTypeConversion3/1 -> AO_2_Ia/1
  Ground3/1 -> DataTypeConversion3/1
  DataTypeConversion4/1 -> AO_3_Ib/1
  Ground4/1 -> DataTypeConversion4/1
  DataTypeConversion5/1 -> AO_4_Ic/1
  Ground5/1 -> DataTypeConversion5/1
  DataTypeConversion6/1 -> AO_5_Rsvl_sin_pos/1
  Ground6/1 -> DataTypeConversion6/1
  DataTypeConversion7/1 -> AO_7_Rsvl_cos_pos/1
  Ground7/1 -> DataTypeConversion7/1
  DataTypeConversion8/1 -> 1_8_Null_AO_trigger/1
  Ground8/1 -> DataTypeConversion8/1
  PWM1A TTL_0/1 -> Terminator1/1
  PWM1B TTL_1/1 -> Terminator2/1
  PWM2A TTL_2/1 -> Terminator3/1
  PWM2B TTL_3/1 -> Terminator4/1
  PWM3A TTL_4/1 -> Terminator5/1
  PWM3B TTL_5/1 -> Terminator6/1
  DataTypeConversion9/1 -> TTL_48_QEP_A_A/1
  Ground9/1 -> DataTypeConversion9/1
  DataTypeConversion10/1 -> TTL_49_QEP_A_B/1
  Ground10/1 -> DataTypeConversion10/1
  DataTypeConversion11/1 -> "TTL_50_QEP_A_I   "/1
  Ground11/1 -> DataTypeConversion11/1
  DataTypeConversion12/1 -> TTL_32_Protocol/1
  Ground12/1 -> DataTypeConversion12/1
  DataTypeConversion13/1 -> TTL_24_AO_trigger_1_8/1
  Ground13/1 -> DataTypeConversion13/1

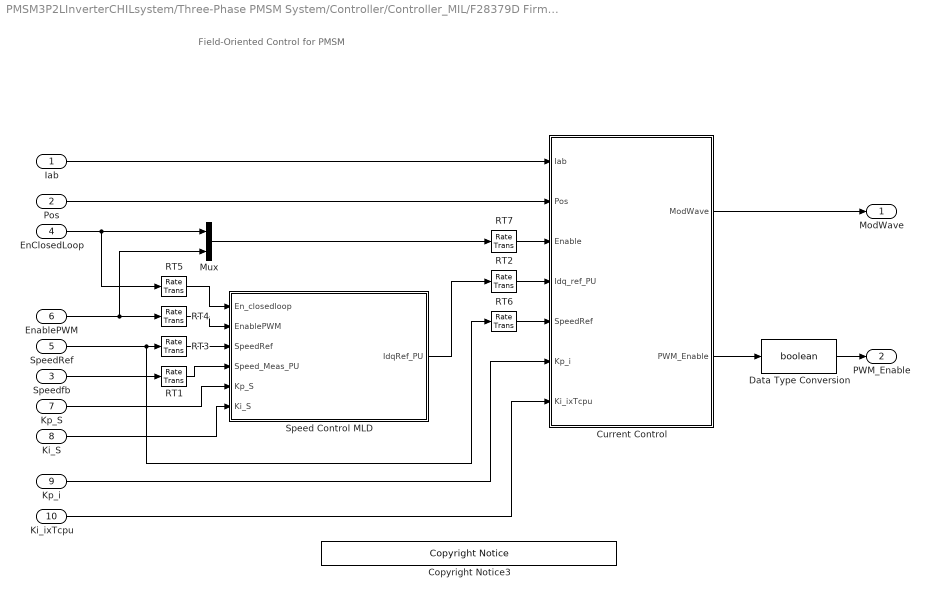
== system PMSM3P2LInverterCHILsystem/Three-Phase PMSM System/Controller/Controller_MIL/F28379D Firmware/Controller Algorithm/FOC ==
  note: Field-Oriented Control for PMSM
  Iab : Inport
  Pos : Inport  Port=2
  Speedfb : Inport  Port=3
  EnClosedLoop : Inport  Port=4
  SpeedRef : Inport  Port=5
  EnablePWM : Inport  Port=6
  Kp_S : Inport  Port=7
  Ki_S : Inport  Port=8
  Kp_i : Inport  Port=9
  Ki_ixTcpu : Inport  Port=10
  Copyright Notice3 : demo_controls/Copyright Notice  year=2020  prod=tic2000
  Current Control : Subsystem  TreatAsAtomicUnit=on
  Data Type Conversion : DataTypeConversion  OutDataTypeStr=boolean  SaturateOnIntegerOverflow=off  RndMeth=Floor
  Mux : Mux  Inputs=2
  RT{1,3..5} (4 alike) : RateTransition  Deterministic=off  OutPortSampleTime=Ts_speed
  RT2 : RateTransition  Deterministic=off
  RT6 : RateTransition  Deterministic=off
  RT7 : RateTransition  Deterministic=off
  Speed Control MLD : Subsystem
  ModWave : Outport
  PWM_Enable : Outport  Port=2
  wires:
  Speed Control MLD/1(IdqRef_PU) -> RT2/1
  EnClosedLoop/1 -> Mux/1, RT5/1
  Speedfb/1 -> RT1/1
  Current Control/2(PWM_Enable) -> Data Type Conversion/1
  EnablePWM/1 -> Mux/2, RT4/1
  Ki_S/1 -> Speed Control MLD/6(Ki_S)
  Current Control/1(ModWave) -> ModWave/1
  Iab/1 -> Current Control/1(Iab)
  Kp_S/1 -> Speed Control MLD/5(Kp_S)
  Pos/1 -> Current Control/2(Pos)
  SpeedRef/1 -> RT6/1, RT3/1
  Mux/1 -> RT7/1
  RT2/1 -> Current Control/4(Idq_ref_PU)
  RT6/1 -> Current Control/5(SpeedRef)
  RT7/1 -> Current Control/3(Enable)
  RT1/1 -> Speed Control MLD/4(Speed_Meas_PU)
  RT3/1 -> Speed Control MLD/3(SpeedRef)
  Data Type Conversion/1 -> PWM_Enable/1
  RT5/1 -> Speed Control MLD/1(En_closedloop)
  RT4/1 -> Speed Control MLD/2(EnablePWM)
  Kp_i/1 -> Current Control/6(Kp_i)
  Ki_ixTcpu/1 -> Current Control/7(Ki_ixTcpu)

== system PMSM3P2LInverterCHILsystem/Three-Phase PMSM System/Controller/Controller_MIL/F28379D Firmware/Controller Algorithm/Speed and Pos Decoder ==
  QEP_Position_Count : Inport
  QEP_Index_Latch : Inport  Port=2
  Offset : Inport  Port=3
  Delay : Delay  DelayLength=1
  IIR Filter : mcbcontrolslib/IIR Filter  VariantControl=Low Pass Filter  VariantSelect=Low-pass  FilterConstantInputType=Specify via dialog  Filter_constant=0.01  InitialOutput=Specify via dialog  InitialOutputValue=0  ExternalReset=none  advancedSettings=off  Ts=50e-6  cutOff_freq=32.1525
  IndexFinder : Subsystem
  Mechanical to Electrical Position : mcbpositiondecoderlib/Mechanical to Electrical Position  PolePairsInputType=Specify via dialog  NrPP=Maxon_645604_Np  selectedRange=Per unit  MechOfstInputType=Input port  mechOffsetIn=0  maxAngleIn=1  InputDataType=single  VariantSelect=floating-point
  NOT : Logic  Operator=NOT  AllPortsSameDT=off  OutDataTypeStr=boolean
  Quadrature Decoder : mcbpositiondecoderlib/Quadrature Decoder  ParameterInputType=off  CountsPerRevInverseDataType=single  EncoderSlitsPerRevolution=Maxon_Mile_Nslits  EncoderCountsPerSlit=4  CounterSize=16 bits  ExternalIndexCount=on  PositionUnit=Per unit  PositionDataType=single
  Speed Measurement : mcbpositiondecoderlib/Speed Measurement  DiscreteStepInput=off  LastDiscreteStepInput=off  PositionUnit=Per unit  PositionScalingDatatype=uint32  SpeedCalculationMode=Time interval for speed calculation  TempSpeedCalculationMode=Time interval for speed calculation  SampleTimeAsync=Ts_CPU  MaximumApplicationSpeed=6000  SpeedResolution=5e-6  DelayLength=20  MaximumMeasurableSpeed=28571.4286  MeasurableSpeedResolution=1.397e-05  SpeedUnit=Per unit based on dialog  TempSpeedUnit=RPM  PerUnitSpeed=PU_System_N_base  SpeedDataType=single
  Theta_e : Outport  VectorParamsAs1DForOutWhenUnconnected=off
  speed : Outport  Port=2  VectorParamsAs1DForOutWhenUnconnected=off
  IndexFound : Outport  Port=3  InitialOutput=0  VectorParamsAs1DForOutWhenUnconnected=off
  wires:
  Mechanical to Electrical Position/1 -> Theta_e/1  "Pos"
  Speed Measurement/1 -> IIR Filter/1
  Quadrature Decoder/1 -> Speed Measurement/1, Mechanical to Electrical Position/1
  QEP_Position_Count/1 -> Quadrature Decoder/1
  Offset/1 -> Mechanical to Electrical Position/2
  IIR Filter/1 -> speed/1
  NOT/1 -> IndexFinder/Enable
  QEP_Index_Latch/1 -> IndexFinder/1(In1), Quadrature Decoder/2
  Delay/1 -> NOT/1
  IndexFinder/1(IndexFound) -> IndexFound/1, Delay/1

== system PMSM3P2LInverterCHILsystem/Three-Phase PMSM System/Controller/Controller_MIL/F28379D Firmware/Controller Algorithm/FOC/Current Control ==
  Iab : Inport
  Pos : Inport  Port=2
  Enable : Inport  Port=3
  Idq_ref_PU : Inport  Port=4
  SpeedRef : Inport  Port=5
  Kp_i : Inport  Port=6
  Ki_ixTcpu : Inport  Port=7
  Control_System : Subsystem
  ModWave : Outport  InitialOutput=0  VectorParamsAs1DForOutWhenUnconnected=off
  PWM_Enable : Outport  Port=2  InitialOutput=0  VectorParamsAs1DForOutWhenUnconnected=off
  wires:
  Idq_ref_PU/1 -> Control_System/4(Idq_ref_PU)  "Idq_ref"
  Pos/1 -> Control_System/2(Pos_PU)  "Pos_PU"
  Enable/1 -> Control_System/3(Enable)
  Iab/1 -> Control_System/1(Iab_meas_PU)  "Iab"
  SpeedRef/1 -> Control_System/5(SpeedRef)
  Control_System/1(ModWave) -> ModWave/1
  Control_System/2(PWM_Enable) -> PWM_Enable/1
  Kp_i/1 -> Control_System/6(Kp_i)
  Ki_ixTcpu/1 -> Control_System/7(Ki_ixTcpu)

== system PMSM3P2LInverterCHILsystem/Three-Phase PMSM System/Controller/Controller_MIL/F28379D Firmware/Controller Algorithm/FOC/Speed Control MLD ==
  En_closedloop : Inport
  EnablePWM : Inport  Port=2
  SpeedRef : Inport  Port=3
  Speed_Meas_PU : Inport  Port=4
  Kp_S : Inport  Port=5
  Ki_S : Inport  Port=6
  AND : Logic  IconShape=distinctive  AllPortsSameDT=off  OutDataTypeStr=boolean
  Id_Ref : Constant  Value=0  OutDataTypeStr=single
  Mux : Mux  Inputs=2
  PI_Controller_Speed : Subsystem
  Speed_Ref_Selector : Subsystem
  IdqRef_PU : Outport  VectorParamsAs1DForOutWhenUnconnected=off
  wires:
  En_closedloop/1 -> PI_Controller_Speed/1(Enable), AND/1
  EnablePWM/1 -> AND/2
  SpeedRef/1 -> Speed_Ref_Selector/2(SpeedCommand)
  AND/1 -> Speed_Ref_Selector/1(Enable)
  Speed_Meas_PU/1 -> PI_Controller_Speed/3(N_fb), Speed_Ref_Selector/3(Speed_Ref_Open)
  Kp_S/1 -> PI_Controller_Speed/4(Kp_S)
  Speed_Ref_Selector/1(Speed_Ref_PU) -> PI_Controller_Speed/2(N_ref)
  Ki_S/1 -> PI_Controller_Speed/5(Ki_S)
  Id_Ref/1 -> Mux/1
  PI_Controller_Speed/1(Iq_ref) -> Mux/2
  Mux/1 -> IdqRef_PU/1

== system PMSM3P2LInverterCHILsystem/Three-Phase PMSM System/Controller/Controller_MIL/F28379D Firmware/Controller Algorithm/Speed and Pos Decoder/IndexFinder ==
  In1 : Inport
  Enable : EnablePort
  AND : Logic  AllPortsSameDT=off  OutDataTypeStr=boolean
  Compare To Constant : simulink/Logic and Bit Operations/Compare To Constant  relop===  const=0  OutDataTypeStr=boolean
  Compare To Constant1 : simulink/Logic and Bit Operations/Compare To Constant  relop=>  const=0  OutDataTypeStr=boolean
  Delay3 : Delay  DelayLength=1
  IndexFound : Outport
  wires:
  In1/1 -> Delay3/1, Compare To Constant1/1
  Compare To Constant1/1 -> AND/2
  Compare To Constant/1 -> AND/1
  Delay3/1 -> Compare To Constant/1
  AND/1 -> IndexFound/1

== system PMSM3P2LInverterCHILsystem/Three-Phase PMSM System/Controller/Controller_MIL/F28379D Firmware/Controller Algorithm/FOC/Current Control/Control_System ==
  Iab_meas_PU : Inport
  Pos_PU : Inport  Port=2
  Enable : Inport  Port=3
  Idq_ref_PU : Inport  Port=4
  SpeedRef : Inport  Port=5
  Kp_i : Inport  Port=6
  Ki_ixTcpu : Inport  Port=7
  Closed Loop Control : Subsystem
  Demux : Demux  Outputs=2
  NOT : Logic  Operator=NOT  IconShape=distinctive  AllPortsSameDT=off  OutDataTypeStr=boolean
  Open Loop Start-Up : Subsystem
  Output Scaling : Subsystem
  Switch : Switch  Criteria=u2 > Threshold  Threshold=0.5  SaturateOnIntegerOverflow=off  InputSameDT=off
  ModWave : Outport
  PWM_Enable : Outport  Port=2
  Idq_debug : Outport  Port=3  VectorParamsAs1DForOutWhenUnconnected=off
  wires:
  Open Loop Start-Up/1(PWM_Duty) -> Switch/3
  Switch/1 -> Output Scaling/1(PWM_Duty)
  Enable/1 -> Demux/1
  Demux/1 -> Closed Loop Control/Enable, Switch/2, NOT/1
  Demux/2 -> [EnablePWM], Open Loop Start-Up/1(<EnablePWM>)
  Iab_meas_PU/1 -> Closed Loop Control/1(Iab_meas_PU)
  Pos_PU/1 -> Closed Loop Control/2(Pos_PU)
  Idq_ref_PU/1 -> Closed Loop Control/3(Idq_ref_PU)  "idqref"
  [EnablePWM] -> Closed Loop Control/4(EnablePWM)
  Closed Loop Control/1(Idq_debug) -> Idq_debug/1
  Closed Loop Control/2(Vabc in PU) -> Switch/1
  Output Scaling/1(ModWave) -> ModWave/1
  Output Scaling/2(PWM_Enable) -> PWM_Enable/1
  [EnablePWM] -> Output Scaling/2(Enable)
  SpeedRef/1 -> Open Loop Start-Up/2(SpeedRef)
  NOT/1 -> Open Loop Start-Up/Enable
  Ki_ixTcpu/1 -> Closed Loop Control/6(Ki_ixTcpu)
  Kp_i/1 -> Closed Loop Control/5(Kp_i)
